simulink model "simulation"  (Simulink 7.9)
settings: Solver=ode1  StartTime=0.0  StopTime=20  FixedStep=0.002  RelTol=1e-3
values from neighbouring files (symbols this model uses):
  A = double(subs(jacobian(F_EOM_Nonlin, states), [states, ctrl_input, design_para], [0, theta_e, 0, 0, 0, 0,F_1_e,F_2_e,beta_1_e,beta_2_e,design_var]))    [Copy_of_EOM.m]    (also in EOM.m = double(subs(jacobian(F_EOM_Nonlin, states), [states, ctrl_in; PID_Tuning.m; wingarea.m = 0.5232)
  B = double(subs(jacobian(F_EOM_Nonlin, ctrl_input), [states, ctrl_input, design_para], [0, theta_e, 0, 0, 0, 0,F_1_e,F_2_e,beta_1_e,beta_2_e,design_var]))    [Copy_of_EOM.m]    (also in EOM.m = double(subs(jacobian(F_EOM_Nonlin, ctrl_input), [states, ctr; PID_Tuning.m)
  C = eye(6)    [Copy_of_EOM.m]    (also in EOM.m; PID_Tuning.m)
  D = zeros(6,4)    [Copy_of_EOM.m]    (also in EOM.m; PID_Tuning.m)
  K = lqr(A, B, Q, R)    [Copy_of_EOM.m]    (also in EOM.m = lqr(Ai, Bi, Q, R))
settings Model: Creator=zhang794  LastModifiedBy=zhang794  ExtModeTrigDuration=5000
settings SolverCC: PositivePriorityOrder=on
settings RTWCC: SystemTargetFile=quarc_win64.tlc  TemplateMakefile=quarc_default_tmf  Description=QUARC Win64 Target  ProcessScript=quarc_win64_make_rtw_hook
settings STFCustomTargetCC: TargetPreCompLibLocation=C:\PROGRA~3\QUARC\lib\2012a\win64\release  CodeReplacementLibrary=ANSI_C  GeneratePreprocessorConditionals=Disable all  CombineOutputUpdateFcns=on  GRTInterface=off  SystemTargetFile=quarc_win64.tlc
settings GRTTargetCC: TargetPreCompLibLocation=C:\PROGRA~3\QUARC\lib\2012a\win64\release  ParMdlRefBuildCompliant=off  CompOptLevelCompliant=off  ConcurrentExecutionCompliant=off  MatFileLogging=off  ExtMode=on  ExtModeMexFile=quarc_comm

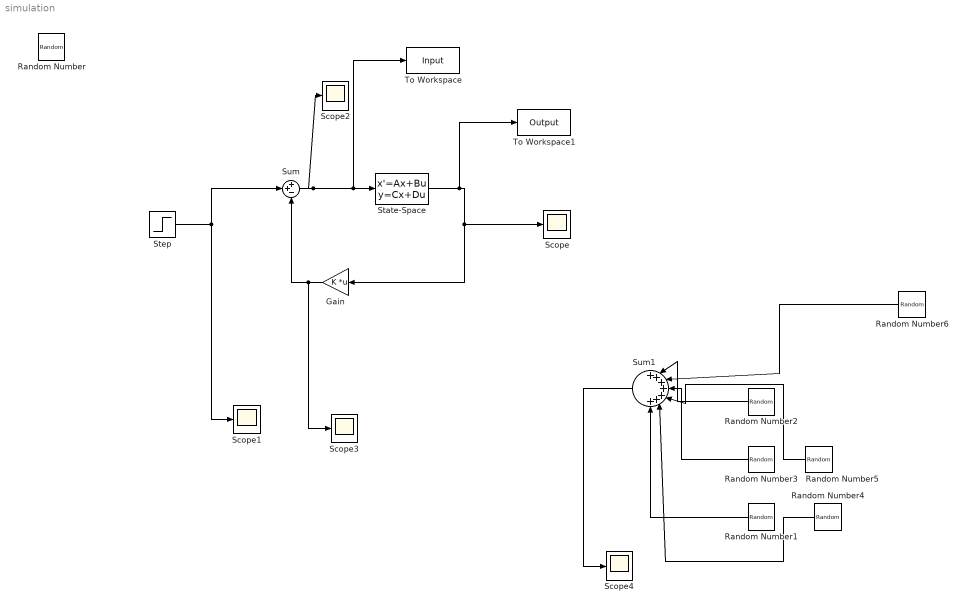
== system simulation ==
  Gain : Gain  Gain=K  Multiplication=Matrix(K*u)
  Random Number : RandomNumber  Mean=[0;0;0;0]  Variance=[0.0905;0.0905;0.0;0.0]  Seed=26  SampleTime=0
  Random Number1 : RandomNumber  Mean=[0;0;0;0;0;0.]  Variance=[0 0 0.0001 0 0 0]  Seed=1363  SampleTime=0
  Random Number2 : RandomNumber  Mean=[0;0;0;0;0;0.]  Variance=[0.0001 0 0 0 0 0]  Seed=2535  SampleTime=0
  Random Number3 : RandomNumber  Mean=[0;0;0;0;0;0.]  Variance=[0 0.0001 0 0 0 0]  Seed=5747  SampleTime=0
  Random Number4 : RandomNumber  Mean=[0;0;0;0;0;0.]  Variance=[0 0 0 0.0033/4 0 0]  Seed=136613  SampleTime=0
  Random Number5 : RandomNumber  Mean=[0;0;0;0;0;0.]  Variance=[0 0 0 0 0.0033/4 0]  Seed=3535  SampleTime=0
  Random Number6 : RandomNumber  Mean=[0;0;0;0;0;0.]  Variance=[0 0 0 0 0 0.0033/4]  Seed=436346  SampleTime=0
  Scope{,1..4} (5 alike) : Scope
      Scope2 settings: TimeRange=2.689618074233458  YMin=-0.6776315789473661  YMax=0.1907894736842128  SaveName=ScopeData2
      Scope3 settings: SaveName=ScopeData3
      Scope4 settings: SaveName=ScopeData4
  State-Space : StateSpace  A=A  B=B  C=C  D=D  X0=[0 0.3 0 0 0 0]
  Step : Step  Time=0  Before=[9;10;0.08;-0.1]  After=[9;9;1;1]  SampleTime=0
  Sum : Sum  Inputs=++-
  Sum1 : Sum  Inputs=+++++++
  To Workspace : ToWorkspace  VariableName=Input  SampleTime=-1  SaveFormat=Structure With Time
  To Workspace1 : ToWorkspace  VariableName=Output  SampleTime=-1  SaveFormat=Structure With Time
  wires:
  Sum/1 -> Scope2/1, State-Space/1, To Workspace/1
  State-Space/1 -> Scope/1, Gain/1, To Workspace1/1
  Step/1 -> Scope1/1, Sum/2
  Gain/1 -> Sum/3, Scope3/1
  Sum1/1 -> Scope4/1
  Random Number2/1 -> Sum1/2
  Random Number6/1 -> Sum1/3
  Random Number3/1 -> Sum1/4
  Random Number5/1 -> Sum1/5
  Random Number4/1 -> Sum1/6
  Random Number1/1 -> Sum1/7
